simulink model "ImaginaryShortTest"  (R2019b)
settings: Solver=ode15s  StartTime=0.0  StopTime=0.01  MaxStep=0.00001  RelTol=1e-3
libraries: fl_lib x7, nesl_utility x4
settings Model: Creator=ykamatan  LastModifiedBy=ykamatan
settings SolverCC: ZeroCrossAlgorithm=Adaptive  SolverResetMethod=Robust
settings DebuggingCC: AlgebraicLoopMsg=none  UnconnectedInputMsg=none  UnconnectedOutputMsg=none  UnconnectedLineMsg=none  SFMachineParentedDataDiag=error
settings ModelReferenceCC: EnableRefExpFcnMdlSchedulingChecks=off
settings RTWCC: Description=Generic Real-Time Target

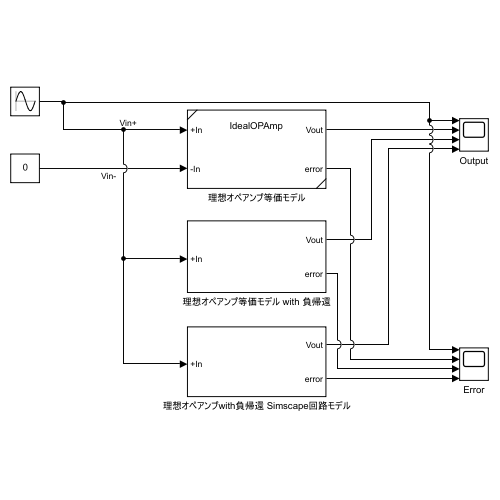
[thumbnail: Simulink's stored preview of the top-level diagram]
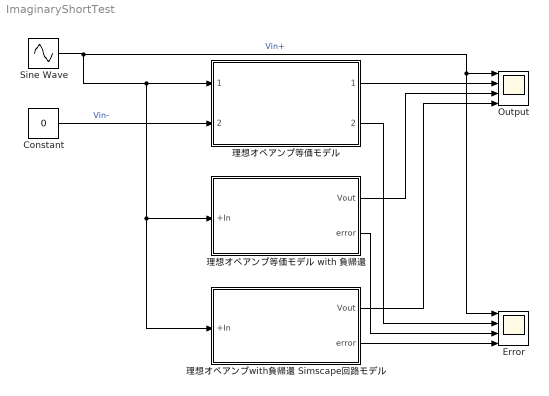
== system ImaginaryShortTest ==
  Constant : Constant  Value=0
  Error : Scope  NumInputPorts=4
  Output : Scope  NumInputPorts=4
  Sine Wave : Sin  Amplitude=3.3  Frequency=2*pi*440  SampleTime=0
  理想オペアンプwith負帰還 Simscape回路モデル : Subsystem
  理想オペアンプ等価モデル : Subsystem  ReferencedSubsystem=IdealOPAmp
  理想オペアンプ等価モデル with 負帰還 : Subsystem
  wires:
  Sine Wave/1 -> 理想オペアンプwith負帰還 Simscape回路モデル/1(+In), 理想オペアンプ等価モデル with 負帰還/1(+In), 理想オペアンプ等価モデル/1, Error/1, Output/1  "Vin+"
  理想オペアンプ等価モデル/1 -> Output/2
  Constant/1 -> 理想オペアンプ等価モデル/2  "Vin-"
  理想オペアンプ等価モデル with 負帰還/1(Vout) -> Output/3
  理想オペアンプwith負帰還 Simscape回路モデル/1(Vout) -> Output/4
  理想オペアンプwith負帰還 Simscape回路モデル/2(error) -> Error/4
  理想オペアンプ等価モデル with 負帰還/2(error) -> Error/3
  理想オペアンプ等価モデル/2 -> Error/2

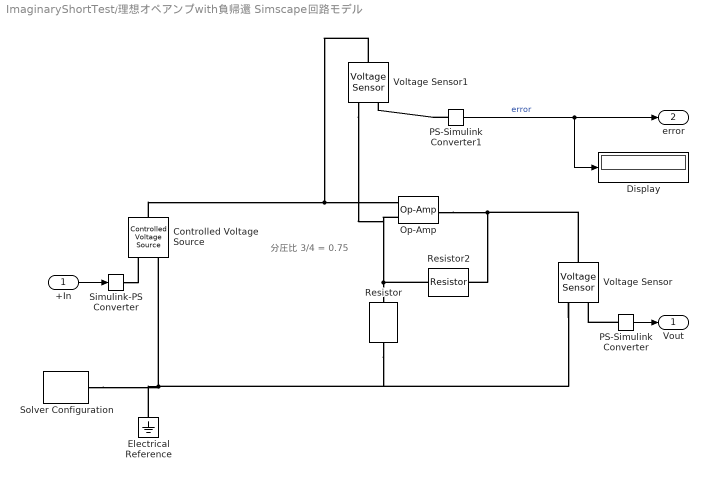
== system ImaginaryShortTest/理想オペアンプwith負帰還 Simscape回路モデル ==
  note: 分圧比 3/4 = 0.75
  +In : Inport
  Controlled Voltage Source : fl_lib/Electrical/Electrical Sources/Controlled Voltage Source
  Display : Display
  Electrical Reference : fl_lib/Electrical/Electrical Elements/Electrical Reference
  Op-Amp : fl_lib/Electrical/Electrical Elements/Op-Amp  outI_specify=off  outI_priority=None  outI=0 A  outI_nominal_specify=off  outI_nominal_unit=A  outI_nominal_value=1
  PS-Simulink Converter : nesl_utility/PS-Simulink Converter  PhysicalDomain=network_engine_domain  SubClassName=ps_output  LeftPortType=input  RightPortType=output  PseudoPeriodic=off  Frequencies=[]  VectorFormat=inherit  Unit=inherit  AffineConversion=off
  PS-Simulink Converter1 : nesl_utility/PS-Simulink Converter  PhysicalDomain=network_engine_domain  SubClassName=ps_output  LeftPortType=input  RightPortType=output  PseudoPeriodic=off  Frequencies=[]  VectorFormat=inherit  Unit=inherit  AffineConversion=off
  Resistor : fl_lib/Electrical/Electrical Elements/Resistor  R=30 MOhm  i_specify=off  i_priority=None  i=0 A  i_nominal_specify=off  i_nominal_unit=A  i_nominal_value=1  v_specify=off  v_priority=None  v=0 V  v_nominal_specify=off  v_nominal_unit=V  v_nominal_value=1
      settings: AttributesFormatString=%<R>%<R_unit>
  Resistor2 : fl_lib/Electrical/Electrical Elements/Resistor  R=10 MOhm  i_specify=off  i_priority=None  i=0 A  i_nominal_specify=off  i_nominal_unit=A  i_nominal_value=1  v_specify=off  v_priority=None  v=0 V  v_nominal_specify=off  v_nominal_unit=V  v_nominal_value=1
      settings: AttributesFormatString=%<R>%<R_unit>
  Simulink-PS Converter : nesl_utility/Simulink-PS Converter  PhysicalDomain=network_engine_domain  SubClassName=ps_input  LeftPortType=input  RightPortType=output  PseudoPeriodic=off  Frequencies=[]  NoiseDistribution=none  NoiseParameters=[]  Unit=1  AffineConversion=off  FilteringAndDerivatives=provide  SimscapeFilterOrder=1  InputFilterTimeConstant=0.001  UdotUserProvided=0
  Solver Configuration : nesl_utility/Solver Configuration  PhysicalDomain=network_engine_domain  SubClassName=solver  LeftPortType=input  RightPortType=generic  Tones=[]  Harmonics=[]  SimulateNoise=off  Profile=off  UseLocalSampling=off  EnableSwitchedLinearOptims=on  FrequencyDomain=off  UseCCode=off  RelTol=0.001  AbsTol=0.001  MinStep=1e-09  ToWorkspace=off  RevertToSquareIcSolve=off  NumHomotopyIterations=100  PhasorMode=off  PhasorModeNumHarmonics=1  ConsistencySolver=NEWTON_XTOL_AFTER_FTOL  IndexReductionMethod=DerivativeReplacement  DoDC=off  ResidualTolerance=1e-09  ConsistencyTolSource=GLOBAL  ConsistencyAbsTol=0.001  ConsistencyRelTol=0.001  ConsistencyTolFactor=0.001  UseLocalSolver=off  LocalSolverChoice=NE_BACKWARD_EULER_ADVANCER  ResolveIndetEquations=on  FunctionEvalNumThread=1  LocalSolverSampleTime=0.001  DoFixedCost=off  MaxNonlinIter=3  MaxModeIter=2  ComputeImpulses=off  ImpulseIterations=2  LinearAlgebra=auto  LinearAlgebraNumThread=0  EquationFormulation=NE_TIME_EF  DelaysMemoryBudget=1024  AutomaticFiltering=on  FilteringTimeConstant=0.001  PartitionStorageMethod=AS_NEEDED  PartitionMemoryBudget=1024  PartitionMethod=ROBUST
  Voltage Sensor : fl_lib/Electrical/Electrical Sensors/Voltage Sensor
  Voltage Sensor1 : fl_lib/Electrical/Electrical Sensors/Voltage Sensor
  Vout : Outport
  error : Outport  Port=2
  wires:
  PS-Simulink Converter/1 -> Vout/1
  +In/1 -> Simulink-PS Converter/1
  PS-Simulink Converter1/1 -> error/1, Display/1  "error"
  connections:
  Resistor2/RConn1 -- Voltage Sensor1/RConn2 -- Op-Amp/LConn2 -- Resistor/LConn1
  Electrical Reference/LConn1 -- Voltage Sensor/RConn2 -- Resistor/RConn1 -- Controlled Voltage Source/RConn2 -- Solver Configuration/RConn1
  Op-Amp/RConn1 -- Voltage Sensor/LConn1 -- Resistor2/LConn1
  Controlled Voltage Source/LConn1 -- Voltage Sensor1/LConn1 -- Op-Amp/LConn1
  PS-Simulink Converter/LConn1 -- Voltage Sensor/RConn1
  Simulink-PS Converter/RConn1 -- Controlled Voltage Source/RConn1
  PS-Simulink Converter1/LConn1 -- Voltage Sensor1/RConn1

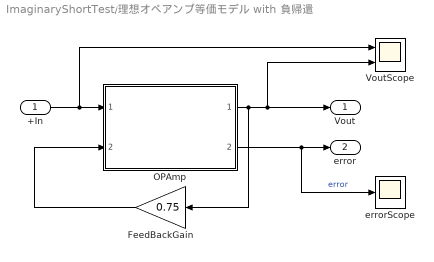
== system ImaginaryShortTest/理想オペアンプ等価モデル with 負帰還 ==
  +In : Inport
  FeedBackGain : Gain  Gain=0.75
  OPAmp : Subsystem  ReferencedSubsystem=IdealOPAmp
  VoutScope : Scope  NumInputPorts=2
  errorScope : Scope
  Vout : Outport
  error : Outport  Port=2
  wires:
  +In/1 -> VoutScope/1, OPAmp/1
  OPAmp/1 -> Vout/1, VoutScope/2, FeedBackGain/1
  FeedBackGain/1 -> OPAmp/2
  OPAmp/2 -> errorScope/1, error/1  "error"
